simulink model "audio_reconstrction"  (R2022b)
settings: Solver=VariableStepAuto  StartTime=0.0  StopTime=10.0  RelTol=1e-3
libraries: dspsnks4 x1, dspvision x1
settings Model: Creator=ECAD-30  LastModifiedBy=ECAD -24

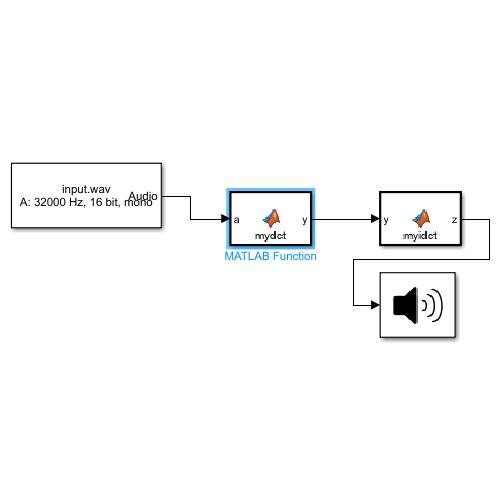
[thumbnail: Simulink's stored preview of the top-level diagram]
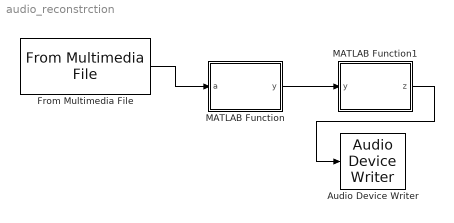
== system audio_reconstrction ==
  Audio Device Writer : dspsnks4/Audio Device Writer  Driver=DirectSound  Device=Default  InheritSampleRate=on  SampleRate=44100  BitDepth=16-bit integer  BufferSize=4096  NumBuffers=10  DefaultOutputChannelMapping=on  OutputChannelMapping=1:2  OutputNumUnderrunSamples=off  DriverIdx=1  DeviceWarnFlag=''
  From Multimedia File : dspvision/From Multimedia File  inputFilename=C:\Users\ECAD -24\Desktop\21UCC125_Lab7\input.wav  readRange=[1 Inf]  loop=on  numPlays=inf  outputStreams=Audio only  videoDataType=single  audioDataType=double  inheritSampleTime=on  userDefinedSampleTime=1/30  noAudioOutput=off  isIntensityVideo=off  fourcc=RGB  colorVideoFormat=Separate color signals  outputEOF=off  dataOrg=Column-major  audioFrameSize=256  computeAudioFrameSize=off  outSamplingMode=Sample based
      settings: LibrarySourceBlock=audiosources/From Multimedia File
  MATLAB Function : MATLAB Function  TreatAsAtomicUnit=on
  MATLAB Function1 : MATLAB Function  TreatAsAtomicUnit=on
  wires:
  From Multimedia File/1 -> MATLAB Function/1(a)
  MATLAB Function/1(y) -> MATLAB Function1/1(y)
  MATLAB Function1/1(z) -> Audio Device Writer/1

== matlab function audio_reconstrction/MATLAB Function ==
  data: a input; y output
function y = mydct(a)
N=256;
w1=1/sqrt(N);
w2=sqrt(2/N);
y=zeros(N,1);
for k=1:N
         if k==1
            w = w1;
         else
            w = w2;
         end 
          temp=0;
          for n=1:N
            temp=temp+(a(n)*cos(pi*(1/(2*N))*((2*n)-1)*(k-1)));
          end
          y(k)=w*temp;
end
end

== matlab function audio_reconstrction/MATLAB Function1 ==
  data: y input; z output
function z  = myidct(y)
N=256;
w1=1/sqrt(N);
w2=sqrt(2/N);
z = zeros(N,1);

for n = 1:N
    temp = 0;
    for k = 1:N
        if(k==1)
            w = w1;
        else
            w = w2;
        end    
        temp = temp + (w*y(k)*cos(pi*(1/(2*N))*((2*n)-1)*(k-1)));
    end 
    z(n)=temp;
end
end
